simulink model "p2_a"  (R2021b)
settings: Solver=VariableStepAuto  StartTime=0.0  StopTime=3  RelTol=1e-3
values from neighbouring files (symbols this model uses):
  c = 0.6811    [hw5_2plot.m]
  c1 = 0.2642    [hw5_2plot.m]
settings Model: Creator=Tomo  LastModifiedBy=Tomo

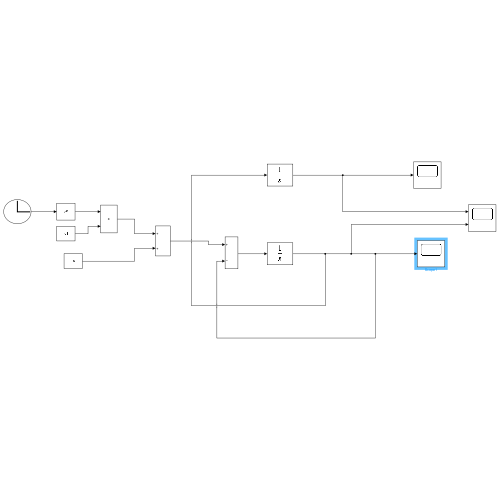
[thumbnail: Simulink's stored preview of the top-level diagram]
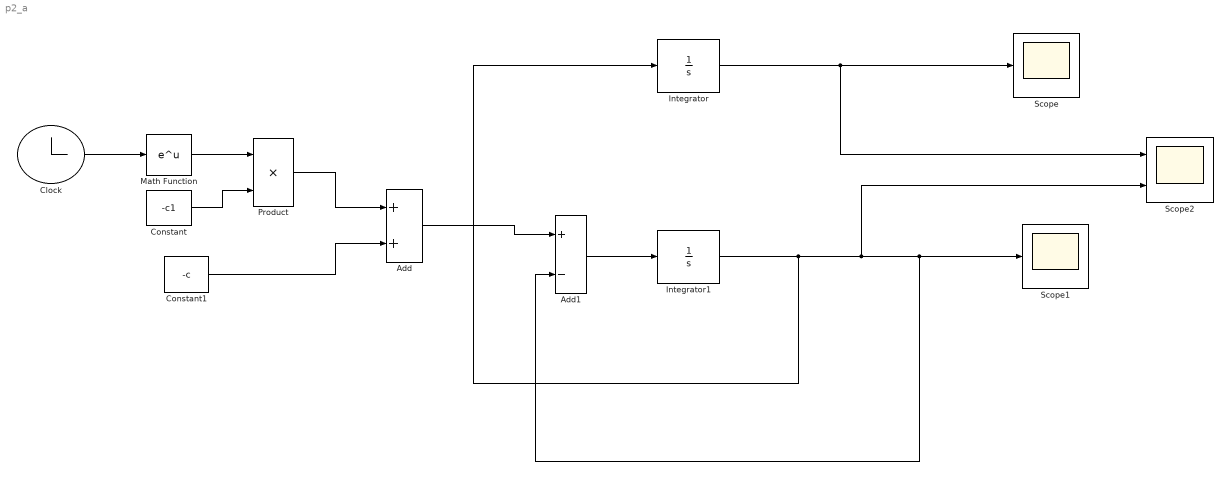
== system p2_a ==
  Add : Sum
  Add1 : Sum  Inputs=+-
  Clock : Clock
      settings: Decimation=100
  Constant : Constant  Value=-c1
  Constant1 : Constant  Value=-c
  Integrator : Integrator
  Integrator1 : Integrator
  Math Function : Math  OutputSignalType=real  SaturateOnIntegerOverflow=on
  Product : Product
  Scope : Scope
  Scope1 : Scope
  Scope2 : Scope  NumInputPorts=2
  wires:
  Integrator/1 -> Scope2/1, Scope/1
  Integrator1/1 -> Scope2/2, Add1/2, Scope1/1, Integrator/1
  Clock/1 -> Math Function/1
  Math Function/1 -> Product/1
  Constant/1 -> Product/2
  Constant1/1 -> Add/2
  Product/1 -> Add/1
  Add/1 -> Add1/1
  Add1/1 -> Integrator1/1
